simulink model "tanques_sim_3"  (R2018a)
settings: Solver=ode45  StartTime=0.0  StopTime=20  RelTol=1e-4
settings Model: Creator=Martin  LastModifiedBy=Alan
settings CodeAppCC: StateflowObjectComments=on

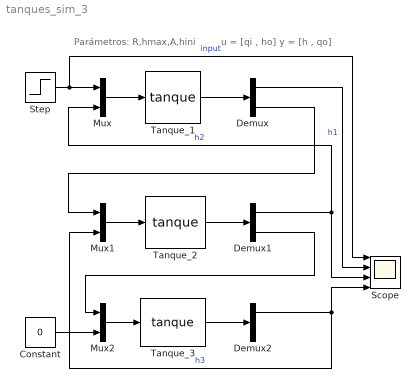
== system tanques_sim_3 ==
  note: u = [qi , ho] y = [h , qo]
  note: Parámetros: R,hmax,A,hini
  Constant : Constant  Value=0
  Demux : Demux  Outputs=2
  Demux1 : Demux  Outputs=2
  Demux2 : Demux  Outputs=2
  Mux : Mux  Inputs=2
  Mux1 : Mux  Inputs=2
  Mux2 : Mux  Inputs=2
  Scope : Scope  NumInputPorts=4
  Step : Step  SampleTime=0
  Tanque_1 : S-Function  FunctionName=tanque  Parameters=0.5,10,2,5  SFunctionDeploymentMode=off  EnableBusSupport=off
  Tanque_2 : S-Function  FunctionName=tanque  Parameters=0.75,10,2,2  SFunctionDeploymentMode=off  EnableBusSupport=off
  Tanque_3 : S-Function  FunctionName=tanque  Parameters=0.75,6,2,0  SFunctionDeploymentMode=off  EnableBusSupport=off
  wires:
  Tanque_1/1 -> Demux/1
  Step/1 -> Mux/1, Scope/1  "input"
  Mux/1 -> Tanque_1/1
  Tanque_2/1 -> Demux1/1
  Demux1/1 -> Scope/3, Mux/2  "h2"
  Demux/2 -> Mux1/1
  Mux1/1 -> Tanque_2/1
  Demux/1 -> Scope/2  "h1"
  Demux1/2 -> Mux2/1
  Mux2/1 -> Tanque_3/1
  Constant/1 -> Mux2/2
  Tanque_3/1 -> Demux2/1
  Demux2/1 -> Mux1/2, Scope/4  "h3"
